simulink subsystem "rocket_model"  (R2022a)
settings: Solver=VariableStepAuto  StartTime=0.0  StopTime=10.0  RelTol=1e-3
undefined symbols (not defined in the file): c, g_x, g_y, L, phi_0, T, x_0, y_0
settings Model: Creator=semen  LastModifiedBy=semen

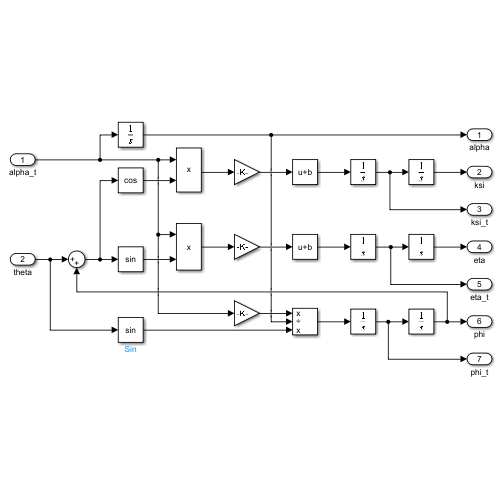
[thumbnail: Simulink's stored preview of the top-level diagram]
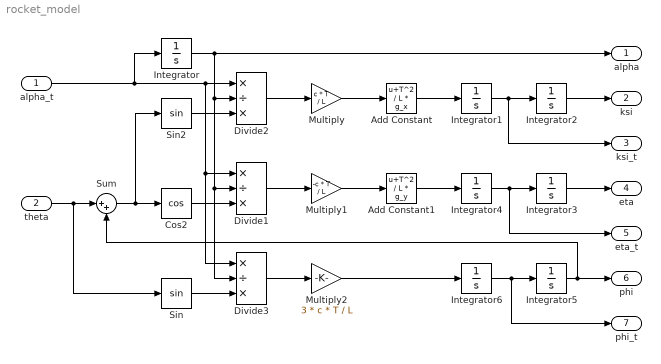
== system rocket_model ==
  alpha_t : Inport
  theta : Inport  Port=2
  Add Constant : Bias  Bias=T^2 / L * g_x  SaturateOnIntegerOverflow=off
  Add Constant1 : Bias  Bias=T^2 / L * g_y  SaturateOnIntegerOverflow=off
  Cos2 : Trigonometry  Operator=cos
  Divide1 : Product  Inputs=*/*
  Divide2 : Product  Inputs=*/*
  Divide3 : Product  Inputs=*/*
  Integrator : Integrator  InitialCondition=1
  Integrator1 : Integrator
  Integrator2 : Integrator  InitialCondition=x_0
  Integrator3 : Integrator  InitialCondition=y_0
  Integrator4 : Integrator
  Integrator5 : Integrator  InitialCondition=phi_0
  Integrator6 : Integrator
  Multiply : Gain  Gain=c * T / L
  Multiply1 : Gain  Gain=-c * T / L
  Multiply2 : Gain  Gain=3 * c * T / L
  Sin : Trigonometry
  Sin2 : Trigonometry
  Sum : Sum  Inputs=|++
  alpha : Outport
  ksi : Outport  Port=2
  ksi_t : Outport  Port=3
  eta : Outport  Port=4
  eta_t : Outport  Port=5
  phi : Outport  Port=6
  phi_t : Outport  Port=7
  wires:
  theta/1 -> Sum/1, Sin/1
  Integrator1/1 -> Integrator2/1, ksi_t/1
  Integrator2/1 -> ksi/1
  Integrator4/1 -> eta_t/1, Integrator3/1
  Integrator3/1 -> eta/1
  Integrator6/1 -> phi_t/1, Integrator5/1
  Integrator5/1 -> phi/1, Sum/2
  Multiply/1 -> Add Constant/1
  Multiply1/1 -> Add Constant1/1
  Sum/1 -> Sin2/1, Cos2/1
  Sin2/1 -> Divide2/3
  Divide2/1 -> Multiply/1
  Cos2/1 -> Divide1/3
  Divide1/1 -> Multiply1/1
  Add Constant/1 -> Integrator1/1
  Add Constant1/1 -> Integrator4/1
  Integrator/1 -> Divide1/2, Divide3/2, Divide2/2, alpha/1
  Sin/1 -> Divide3/3
  alpha_t/1 -> Integrator/1, Divide1/1, Divide3/1, Divide2/1
  Divide3/1 -> Multiply2/1
  Multiply2/1 -> Integrator6/1
